simulink model "DCMotor_Electrical"  (R2016a)
settings: Solver=VariableStepAuto  StartTime=0.0  StopTime=10.0  RelTol=1e-3
libraries: fl_lib x20, nesl_utility x11
settings Model: Creator=kkfrk  LastModifiedBy=kkfrk

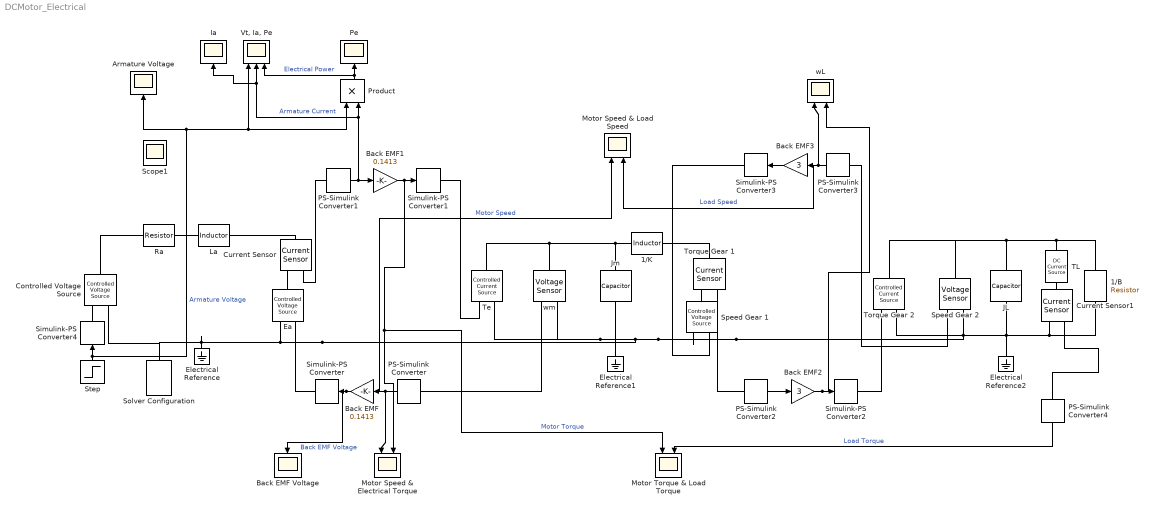
== system DCMotor_Electrical ==
  1/B : fl_lib/Electrical/Electrical Elements/Resistor  R=1/(0.5E-3) Ohm  i_specify=off  i_priority=None  i=0 A  v_specify=off  v_priority=None  v=0 V
  1/K : fl_lib/Electrical/Electrical Elements/Inductor  l=1/8 H  r=0 Ohm  g=1e-9 1/Ohm  i_specify=off  i_priority=None  i=0 A  v_specify=off  v_priority=None  v=0 V  i_L_specify=off  i_L_priority=High  i_L=0 A
  Armature Voltage : Scope
  Back EMF : Gain  Gain=0.1413
  Back EMF Voltage : Scope
  Back EMF1 : Gain  Gain=0.1413
  Back EMF2 : Gain  Gain=3
  Back EMF3 : Gain  Gain=3
  Controlled Voltage Source : fl_lib/Electrical/Electrical Sources/Controlled Voltage Source
  Current Sensor : fl_lib/Electrical/Electrical Sensors/Current Sensor
  Current Sensor1 : fl_lib/Electrical/Electrical Sensors/Current Sensor
  Ea : fl_lib/Electrical/Electrical Sources/Controlled Voltage Source
  Electrical Reference : fl_lib/Electrical/Electrical Elements/Electrical Reference
  Electrical Reference1 : fl_lib/Electrical/Electrical Elements/Electrical Reference
  Electrical Reference2 : fl_lib/Electrical/Electrical Elements/Electrical Reference
  Ia : Scope
  JL : fl_lib/Electrical/Electrical Elements/Capacitor  c=9000e-7 F  r=0 Ohm  g=0 1/Ohm  i_specify=off  i_priority=None  i=0 A  v_specify=off  v_priority=None  v=0 V  vc_specify=off  vc_priority=High  vc=0 V
  Jm : fl_lib/Electrical/Electrical Elements/Capacitor  c=6355e-7 F  r=0 Ohm  g=0 1/Ohm  i_specify=off  i_priority=None  i=0 A  v_specify=off  v_priority=None  v=0 V  vc_specify=off  vc_priority=High  vc=0 V
  La : fl_lib/Electrical/Electrical Elements/Inductor  l=1.3e-3 H  r=0 Ohm  g=1e-9 1/Ohm  i_specify=off  i_priority=None  i=0 A  v_specify=off  v_priority=None  v=0 V  i_L_specify=off  i_L_priority=High  i_L=0 A
  Motor Speed & Electrical Torque : Scope  NumInputPorts=2
  Motor Speed & Load Speed : Scope  NumInputPorts=2
  Motor Torque & Load Torque : Scope  NumInputPorts=2
  PS-Simulink Converter{,1..4} (5 alike) : nesl_utility/PS-Simulink Converter  PhysicalDomain=network_engine_domain  SubClassName=ps_output  LeftPortType=input  RightPortType=output  PseudoPeriodic=off  Frequencies=[]  Unit=1  AffineConversion=off
  Pe : Scope
  Product : Product
  Ra : fl_lib/Electrical/Electrical Elements/Resistor  R=0.7 Ohm  i_specify=off  i_priority=None  i=0 A  v_specify=off  v_priority=None  v=0 V
  Simulink-PS Converter{,1..4} (5 alike) : nesl_utility/Simulink-PS Converter  PhysicalDomain=network_engine_domain  SubClassName=ps_input  LeftPortType=input  RightPortType=output  PseudoPeriodic=off  Frequencies=[]  NoiseDistribution=none  NoiseParameters=[]  Unit=1  AffineConversion=off  InputFiltering=off  SimscapeFilterOrder=1  InputFilterTimeConstant=0.001  UdotUserProvided=1
  Solver Configuration : nesl_utility/Solver Configuration  PhysicalDomain=network_engine_domain  SubClassName=solver  LeftPortType=input  RightPortType=generic  Accelerate=off  Tones=[]  Harmonics=[]  SimulateNoise=off  Profile=off  UseLocalSampling=off  EnableSwitchedLinearOptims=on  FrequencyDomain=off  UseCCode=off  RelTol=0.001  AbsTol=1e-06  MinStep=1e-09  ToWorkspace=off  RevertToSquareIcSolve=off  NumHomotopyIterations=100  PhasorMode=off  PhasorModeNumHarmonics=1  OverrideAbsTol=off  DoDC=off  ResidualTolerance=1e-09  UseLocalSolver=off  LocalSolverChoice=NE_BACKWARD_EULER_ADVANCER  LocalSolverSampleTime=0.001  DoFixedCost=off  MaxNonlinIter=3  MaxModeIter=2  LinearAlgebra=Sparse  DelaysMemoryBudget=1024  AutomaticFiltering=on  FilteringTimeConstant=0.001
  Speed Gear 2 : fl_lib/Electrical/Electrical Sensors/Voltage Sensor
  Speed Gear 1 : fl_lib/Electrical/Electrical Sources/Controlled Voltage Source
  Step : Step  Time=5  Before=48  After=24  SampleTime=0
  TL : fl_lib/Electrical/Electrical Sources/DC Current Source  i0=1.5 A
  Te : fl_lib/Electrical/Electrical Sources/Controlled Current Source
  Torque Gear 2 : fl_lib/Electrical/Electrical Sources/Controlled Current Source
  Torque Gear 1 : fl_lib/Electrical/Electrical Sensors/Current Sensor
  "Vt, Ia, Pe" : Scope  NumInputPorts=3
  wL : Scope  NumInputPorts=2
  wm : fl_lib/Electrical/Electrical Sensors/Voltage Sensor
  Scope1 : Scope
  wires:
  PS-Simulink Converter/1 -> Motor Speed & Load Speed/1, Motor Speed & Electrical Torque/1, Back EMF/1  "Motor Speed"
  Back EMF/1 -> Back EMF Voltage/1, Simulink-PS Converter/1  "Back EMF Voltage"
  PS-Simulink Converter1/1 -> Back EMF1/1, Ia/1, "Vt, Ia, Pe"/2, Product/2  "Armature Current"
  Back EMF1/1 -> Motor Torque & Load Torque/1, Motor Speed & Electrical Torque/2, Simulink-PS Converter1/1  "Motor Torque"
  PS-Simulink Converter2/1 -> Back EMF2/1
  Back EMF2/1 -> wL/2, Simulink-PS Converter2/1
  PS-Simulink Converter3/1 -> Motor Speed & Load Speed/2, wL/1, Back EMF3/1  "Load Speed"
  Back EMF3/1 -> Simulink-PS Converter3/1
  Step/1 -> Product/1, "Vt, Ia, Pe"/1, Armature Voltage/1, Simulink-PS Converter4/1  "Armature Voltage"
  Product/1 -> "Vt, Ia, Pe"/3, Pe/1  "Electrical Power"
  PS-Simulink Converter4/1 -> Motor Torque & Load Torque/2  "Load Torque"
  connections:
  Current Sensor/RConn2 -- Ea/LConn1
  La/RConn1 -- Current Sensor/LConn1
  Ra/RConn1 -- La/LConn1
  1/B/RConn1 -- Current Sensor1/RConn2 -- Electrical Reference1/LConn1 -- Jm/RConn1 -- wm/RConn2 -- Te/RConn2 -- Controlled Voltage Source/RConn2 -- Solver Configuration/RConn1 -- Electrical Reference/LConn1 -- Ea/RConn2 -- Speed Gear 1/RConn2 -- Torque Gear 2/RConn2 -- Speed Gear 2/RConn2 -- JL/RConn1 -- Electrical Reference2/LConn1
  Te/LConn1 -- wm/LConn1 -- Jm/LConn1 -- 1/K/LConn1
  wm/RConn1 -- PS-Simulink Converter/LConn1
  Simulink-PS Converter/RConn1 -- Ea/RConn1
  Current Sensor/RConn1 -- PS-Simulink Converter1/LConn1
  Simulink-PS Converter1/RConn1 -- Te/RConn1
  JL/LConn1 -- Torque Gear 2/LConn1 -- Speed Gear 2/LConn1 -- TL/RConn1 -- 1/B/LConn1
  Torque Gear 1/RConn2 -- Speed Gear 1/LConn1
  1/K/RConn1 -- Torque Gear 1/LConn1
  Torque Gear 1/RConn1 -- PS-Simulink Converter2/LConn1
  Simulink-PS Converter2/RConn1 -- Torque Gear 2/RConn1
  Speed Gear 2/RConn1 -- PS-Simulink Converter3/LConn1
  Simulink-PS Converter3/RConn1 -- Speed Gear 1/RConn1
  Controlled Voltage Source/LConn1 -- Ra/LConn1
  Simulink-PS Converter4/RConn1 -- Controlled Voltage Source/RConn1
  Current Sensor1/LConn1 -- TL/LConn1
  Current Sensor1/RConn1 -- PS-Simulink Converter4/LConn1
